simulink model "LandingGear"  (R2016a)
settings: Solver=ode3  StartTime=0.0  StopTime=120  FixedStep=0.1  MaxStep=0.1  RelTol=1e-3
InitFcn:
  | SetConstants
StopFcn:
  | ProcessResults
libraries: LandingGearLibrary x11
settings Model: Creator=sj3-wright  LastModifiedBy=sjm2-skilling
settings DataIOCC: LimitDataPoints=on  SaveFormat=Array
settings DebuggingCC: SolverPrmCheckMsg=warning  SignalLabelMismatchMsg=error
settings HardwareCC: ProdBitPerPointer=32  ProdLargestAtomicFloat=None  ProdIntDivRoundTo=Undefined  ProdEndianess=Unspecified  ProdWordSize=32  ProdHWDeviceType=32-bit Generic
settings ModelReferenceCC: PropagateSignalLabelsOutOfModel=off
settings ConfigComp: CovModelRefEnable=Off  CovSFcnEnable=off

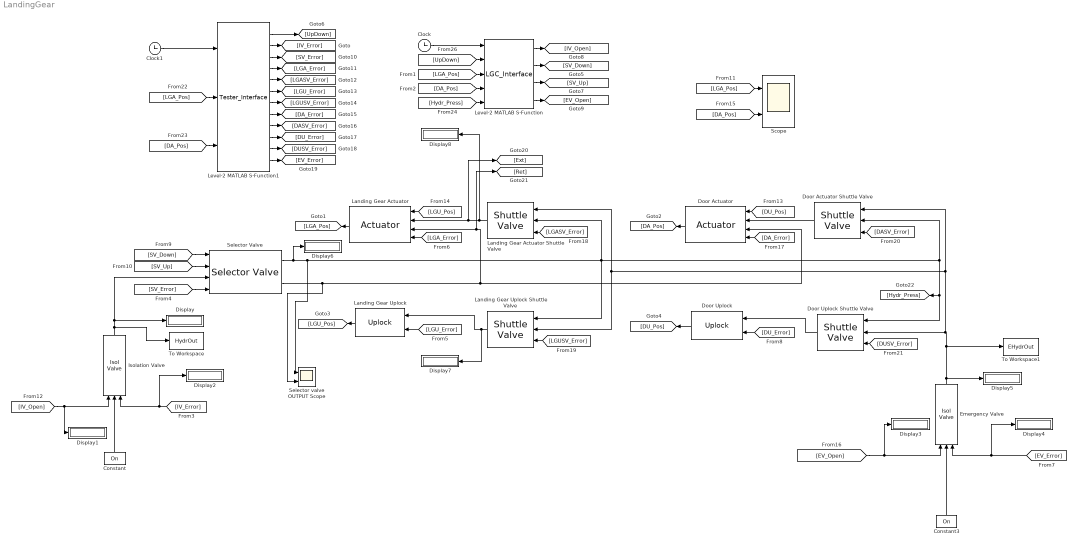
== system LandingGear ==
  Clock : Clock
  Clock1 : Clock
  Constant : Constant  Value=On
  Constant3 : Constant  Value=On
  Display{,1..8} (9 alike) : Display
  Door Actuator : LandingGearLibrary/Actuator
  Door Uplock : LandingGearLibrary/Uplock
  Door Actuator Shuttle Valve : LandingGearLibrary/Shuttle Valve
  Door Uplock Shuttle Valve : LandingGearLibrary/Shuttle Valve
  Emergency Valve : LandingGearLibrary/Isol Valve
  Isolation Valve : LandingGearLibrary/Isol Valve
  Landing Gear Actuator : LandingGearLibrary/Actuator
  Landing Gear Uplock : LandingGearLibrary/Uplock
  Landing Gear Actuator Shuttle Valve : LandingGearLibrary/Shuttle Valve
  Landing Gear Uplock Shuttle Valve : LandingGearLibrary/Shuttle Valve
  Level-2 MATLAB S-Function : M-S-Function  FunctionName=LGC_Interface
  Level-2 MATLAB S-Function1 : M-S-Function  FunctionName=Tester_Interface
  Scope : Scope  NumInputPorts=2
  Selector Valve : LandingGearLibrary/Selector Valve
  "Selector valve OUTPUT Scope " : Scope  NumInputPorts=2
  To Workspace : ToWorkspace  VariableName=HydrOut  SaveFormat=Structure With Time  SampleTime=-1
  To Workspace1 : ToWorkspace  VariableName=EHydrOut  SaveFormat=Structure With Time  SampleTime=-1
  wires:
  Constant/1 -> Isolation Valve/2
  [IV_Open] -> Display1/1, Isolation Valve/1
  Isolation Valve/1 -> To Workspace/1, Display/1, Selector Valve/3
  Landing Gear Actuator/1 -> [LGA_Pos]
  Selector Valve/1 -> Display6/1, "Selector valve OUTPUT Scope "/1, Landing Gear Actuator Shuttle Valve/2, Landing Gear Uplock Shuttle Valve/1, [Hydr_Press], Door Uplock Shuttle Valve/1, Door Actuator Shuttle Valve/2
  Constant3/1 -> Emergency Valve/2
  [EV_Open] -> Display3/1, Emergency Valve/1
  Emergency Valve/1 -> To Workspace1/1, Door Uplock Shuttle Valve/2, Door Actuator Shuttle Valve/1, Landing Gear Uplock Shuttle Valve/2, Landing Gear Actuator Shuttle Valve/1, Display5/1
  Landing Gear Uplock/1 -> [LGU_Pos]
  Door Uplock/1 -> [DU_Pos]
  [DA_Pos] -> Level-2 MATLAB S-Function/4
  [LGA_Pos] -> Level-2 MATLAB S-Function/3
  [SV_Down] -> Selector Valve/1
  [SV_Up] -> Selector Valve/2
  Landing Gear Actuator Shuttle Valve/1 -> Display8/1, [Ext], Landing Gear Actuator/2
  [LGU_Pos] -> Landing Gear Actuator/1
  Level-2 MATLAB S-Function/4 -> [EV_Open]
  Level-2 MATLAB S-Function/3 -> [SV_Up]
  Level-2 MATLAB S-Function/1 -> [IV_Open]
  Level-2 MATLAB S-Function/2 -> [SV_Down]
  Door Actuator/1 -> [DA_Pos]
  [DU_Pos] -> Door Actuator/1
  Door Actuator Shuttle Valve/1 -> Door Actuator/2
  Selector Valve/2 -> "Selector valve OUTPUT Scope "/2, [Ret], Landing Gear Actuator/3, Door Actuator/3
  Clock/1 -> Level-2 MATLAB S-Function/1
  [IV_Error] -> Display2/1, Isolation Valve/3
  [SV_Error] -> Selector Valve/4
  [LGA_Error] -> Landing Gear Actuator/4
  [EV_Error] -> Display4/1, Emergency Valve/3
  [DA_Error] -> Door Actuator/4
  [LGASV_Error] -> Landing Gear Actuator Shuttle Valve/3
  [LGUSV_Error] -> Landing Gear Uplock Shuttle Valve/3
  [DASV_Error] -> Door Actuator Shuttle Valve/3
  [DUSV_Error] -> Door Uplock Shuttle Valve/3
  Clock1/1 -> Level-2 MATLAB S-Function1/1
  Level-2 MATLAB S-Function1/2 -> [IV_Error]
  Level-2 MATLAB S-Function1/1 -> [UpDown]
  Level-2 MATLAB S-Function1/3 -> [SV_Error]
  Level-2 MATLAB S-Function1/4 -> [LGA_Error]
  Level-2 MATLAB S-Function1/5 -> [LGASV_Error]
  Level-2 MATLAB S-Function1/6 -> [LGU_Error]
  Level-2 MATLAB S-Function1/7 -> [LGUSV_Error]
  Level-2 MATLAB S-Function1/8 -> [DA_Error]
  Level-2 MATLAB S-Function1/9 -> [DASV_Error]
  Level-2 MATLAB S-Function1/10 -> [DU_Error]
  Level-2 MATLAB S-Function1/11 -> [DUSV_Error]
  Level-2 MATLAB S-Function1/12 -> [EV_Error]
  [UpDown] -> Level-2 MATLAB S-Function/2
  [LGA_Pos] -> Level-2 MATLAB S-Function1/2
  [DA_Pos] -> Level-2 MATLAB S-Function1/3
  [LGA_Pos] -> Scope/1
  [DA_Pos] -> Scope/2
  [Hydr_Press] -> Level-2 MATLAB S-Function/5
  [DU_Error] -> Door Uplock/2
  Door Uplock Shuttle Valve/1 -> Door Uplock/1
  [LGU_Error] -> Landing Gear Uplock/2
  Landing Gear Uplock Shuttle Valve/1 -> Display7/1, Landing Gear Uplock/1
